simulink model "uavsim_trim"  (R2015a)
settings: Solver=ode45  StartTime=0.0  StopTime=10.0  RelTol=1e-3
undefined symbols (not defined in the file or in its folder): forces_moments, UAV
settings Model: Creator=User  LastModifiedBy=User

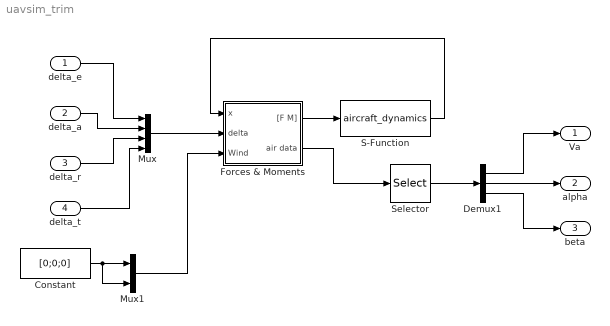
== system uavsim_trim ==
  delta_e : Inport
  delta_a : Inport  Port=2
  delta_r : Inport  Port=3
  delta_t : Inport  Port=4
  Constant : Constant  Value=[0;0;0]
  Demux1 : Demux  Outputs=3
  Forces & Moments : Subsystem
  Mux : Mux
  Mux1 : Mux  Inputs=2
  S-Function : S-Function  FunctionName=aircraft_dynamics  Parameters=UAV
  Selector : Selector  InputPortWidth=6  Indices=[1 2 3]
  Va : Outport
  alpha : Outport  Port=2
  beta : Outport  Port=3
  wires:
  delta_e/1 -> Mux/1
  delta_a/1 -> Mux/2
  delta_r/1 -> Mux/3
  delta_t/1 -> Mux/4
  Mux/1 -> Forces & Moments/2(delta)
  Demux1/2 -> alpha/1
  Constant/1 -> Mux1/2, Mux1/1
  Mux1/1 -> Forces & Moments/3(Wind)
  Forces & Moments/1("[F M]") -> S-Function/1
  S-Function/1 -> Forces & Moments/1(x)
  Forces & Moments/2(air data) -> Selector/1
  Selector/1 -> Demux1/1
  Demux1/3 -> beta/1
  Demux1/1 -> Va/1

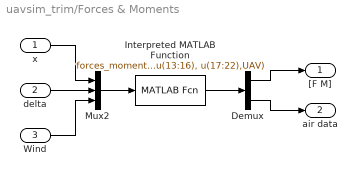
== system uavsim_trim/Forces & Moments ==
  x : Inport
  delta : Inport  Port=2
  Wind : Inport  Port=3
  Demux : Demux  Outputs=[6;6]
  Interpreted MATLAB Function : MATLABFcn  MATLABFcn=forces_moments(u(1:12), u(13:16), u(17:22),UAV)  OutputDimensions=12
  Mux2 : Mux  Inputs=3
  "[F M]" : Outport
  air data : Outport  Port=2
  wires:
  Mux2/1 -> Interpreted MATLAB Function/1
  delta/1 -> Mux2/2
  Wind/1 -> Mux2/3
  x/1 -> Mux2/1
  Demux/2 -> air data/1
  Interpreted MATLAB Function/1 -> Demux/1
  Demux/1 -> "[F M]"/1
